simulink model "EmagFieldSim"  (R2023b)
settings: Solver=VariableStepAuto  StartTime=0.0  StopTime=24670  RelTol=1e-3
values from neighbouring files (symbols this model uses):
  dyear = decyear('20-may-2024','dd-mmm-yyyy')    [Bdot_Controller.m]
  phi = 98*pi/180    (= 1.71042266695)    [Bdot_Controller.m]
undefined symbols (not defined in the file or in its folder): WMM2020
libraries: simulink x1, aerolibgravity2 x1
settings Model: Creator=bogas  LastModifiedBy=bogas

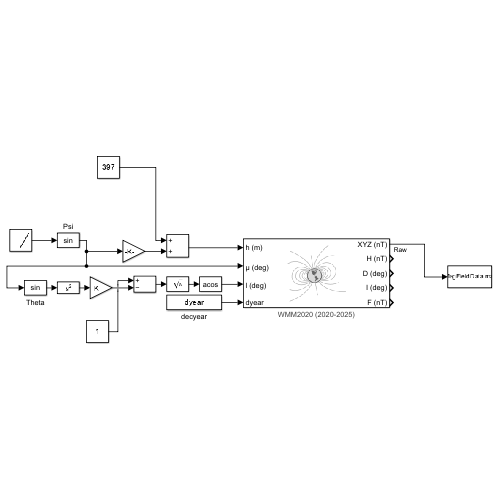
[thumbnail: Simulink's stored preview of the top-level diagram]
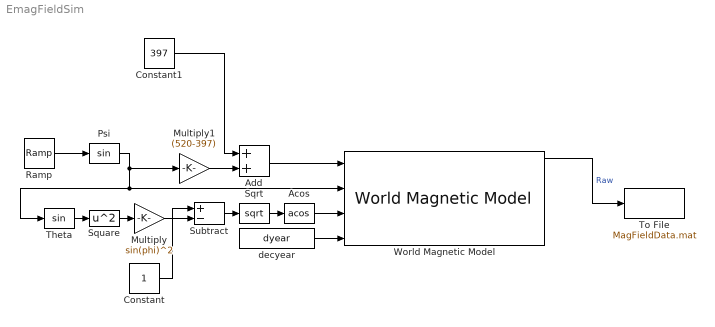
== system EmagFieldSim ==
  Acos : Trigonometry  Operator=acos
  Add : Sum
  Constant : Constant
  Constant1 : Constant  Value=397
  Multiply : Gain  Gain=sin(phi)^2
  Multiply1 : Gain  Gain=(520-397)
  Psi : Trigonometry
  Ramp : simulink/Sources/Ramp  slope=1  start=0  InitialOutput=0
  Sqrt : Sqrt
  Square : Math  Operator=square
  Subtract : Sum  Inputs=+-
  Theta : Trigonometry
  To File : ToFile  Filename=MagFieldData.mat  MatrixName=XYZ  SaveFormat=Timeseries
  World Magnetic Model : aerolibgravity2/World Magnetic Model  model=WMM2020 (2020-2025)  customFile='WMM2020.COF'  units=Metric (MKS)  time_in=on  month=January  day=1  year=2020  action=Error  h_out=on  dec_out=on  inc_out=on  ti_out=on
  decyear : Constant  Value=dyear
  wires:
  World Magnetic Model/1 -> To File/1  "Raw"
  Multiply1/1 -> Add/2
  Acos/1 -> World Magnetic Model/3
  decyear/1 -> World Magnetic Model/4
  Add/1 -> World Magnetic Model/1
  Multiply/1 -> Subtract/2
  Subtract/1 -> Sqrt/1
  Constant/1 -> Subtract/1
  Theta/1 -> Square/1
  Constant1/1 -> Add/1
  Square/1 -> Multiply/1
  Ramp/1 -> Psi/1
  Psi/1 -> Multiply1/1, Theta/1, World Magnetic Model/2
  Sqrt/1 -> Acos/1
